simulink model "inv_pendel4"  (Simulink 4.00)
settings: Solver=ode45  StartTime=0.0  StopTime=10.0  MaxStep=0.01  RelTol=1e-3
values from neighbouring files (symbols this model uses):
  g = 9.89    [inv_pendel_1.m]    (also in inv_pendel_2.m; inv_pendel_3.m; inv_pendel_4.m)
  K = place(a,b,p)    [inv_pendel_2.m]    (also in inv_pendel_3.m; inv_pendel_4.m; zeitdiskret_1.m = [1,0;10,1])
  l = 0.75    [inv_pendel_1.m]    (also in inv_pendel_2.m; inv_pendel_3.m; inv_pendel_4.m)
  M = 5    [inv_pendel_1.m]    (also in inv_pendel_2.m; inv_pendel_3.m; inv_pendel_4.m)
  m = 0.5    [inv_pendel_1.m]    (also in inv_pendel_2.m; inv_pendel_3.m; inv_pendel_4.m; mikrofon1.m = 0.001)
libraries: cstblocks x2
settings Model: LastModifiedBy=Administrator  BlockReductionOpt=off

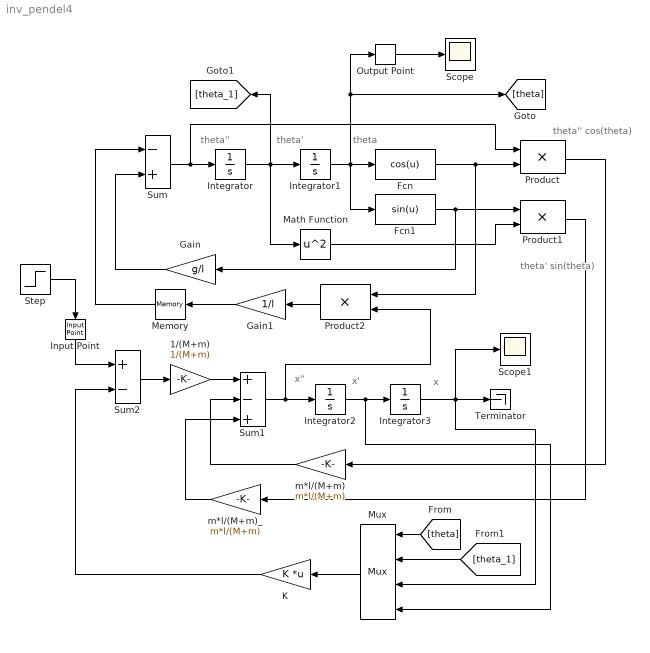
== system inv_pendel4 ==
  note: theta''
  note: theta'
  note: theta
  note: theta'' cos(theta)
  note: theta' sin(theta)
  note: x''
  note: x'
  note: x
  1/(M+m) : Gain  Gain=1/(M+m)  Multiplication=Element-wise(K.*u)  SaturateOnIntegerOverflow=on
  Fcn : Fcn  Expr=cos(u)
  Fcn1 : Fcn  Expr=sin(u)
  Gain : Gain  Orientation=left  Gain=g/l  Multiplication=Element-wise(K.*u)  SaturateOnIntegerOverflow=on
  Gain1 : Gain  Orientation=left  Gain=1/l  Multiplication=Element-wise(K.*u)  SaturateOnIntegerOverflow=on
  Input Point : cstblocks/Input Point  Orientation=down
  Integrator : Integrator  ExternalReset=none  InitialConditionSource=internal  InitialCondition=0  LimitOutput=off  UpperSaturationLimit=inf  LowerSaturationLimit=-inf  ShowSaturationPort=off  ShowStatePort=off  AbsoluteTolerance=auto
  Integrator1 : Integrator  ExternalReset=none  InitialConditionSource=internal  InitialCondition=0.2  LimitOutput=off  UpperSaturationLimit=inf  LowerSaturationLimit=-inf  ShowSaturationPort=off  ShowStatePort=off  AbsoluteTolerance=auto
  Integrator2 : Integrator  ExternalReset=none  InitialConditionSource=internal  InitialCondition=0  LimitOutput=off  UpperSaturationLimit=inf  LowerSaturationLimit=-inf  ShowSaturationPort=off  ShowStatePort=off  AbsoluteTolerance=auto
  Integrator3 : Integrator  ExternalReset=none  InitialConditionSource=internal  InitialCondition=0  LimitOutput=off  UpperSaturationLimit=inf  LowerSaturationLimit=-inf  ShowSaturationPort=off  ShowStatePort=off  AbsoluteTolerance=auto
  K : Gain  Orientation=left  Gain=K  Multiplication=Matrix(K*u)  SaturateOnIntegerOverflow=on
  Math Function : Math  Operator=square  OutputSignalType=auto
  Memory : Memory  Orientation=left  X0=0  InheritSampleTime=off
  Mux : Mux  Orientation=left  Inputs=4
      settings: DisplayOption=none
  Output Point : cstblocks/Output Point
  Product : Product  Inputs=2  Multiplication=Element-wise(.*)  SaturateOnIntegerOverflow=on
  Product1 : Product  Inputs=2  Multiplication=Element-wise(.*)  SaturateOnIntegerOverflow=on
  Product2 : Product  Orientation=left  Inputs=2  Multiplication=Element-wise(.*)  SaturateOnIntegerOverflow=on
  Scope : Scope
      settings: TimeRange=auto  YMin=-1  YMax=1  SaveToWorkspace=off  SaveName=ScopeData  MaxDataPoints=5000
  Scope1 : Scope
      settings: TimeRange=auto  YMin=-1  YMax=4  SaveToWorkspace=off  MaxDataPoints=5000
  Step : Step  Time=0  Before=0  After=1  SampleTime=0
  Sum : Sum  Inputs=-+  SaturateOnIntegerOverflow=on
  Sum1 : Sum  Inputs=+-+  SaturateOnIntegerOverflow=on
  Sum2 : Sum  Inputs=+-  SaturateOnIntegerOverflow=on
  Terminator : Terminator
  m*l/(M+m) : Gain  Orientation=left  Gain=m*l/(M+m)  Multiplication=Element-wise(K.*u)  SaturateOnIntegerOverflow=on
  m*l/(M+m)_ : Gain  Orientation=left  Gain=m*l/(M+m)  Multiplication=Element-wise(K.*u)  SaturateOnIntegerOverflow=on
  wires:
  Sum/1 -> Integrator/1, Product/1
  Integrator/1 -> Integrator1/1, [theta_1], Math Function/1
  Integrator1/1 -> Fcn1/1, Fcn/1, [theta], Output Point/1
  Fcn/1 -> Product2/1, Product/2
  Fcn1/1 -> Product1/1, Gain/1
  Product/1 -> m*l/(M+m)/1
  Gain/1 -> Sum/2
  Product2/1 -> Gain1/1
  Gain1/1 -> Memory/1
  Sum1/1 -> Integrator2/1, Product2/2
  Integrator2/1 -> Integrator3/1, Mux/4
  1/(M+m)/1 -> Sum1/1
  m*l/(M+m)/1 -> Sum1/2
  m*l/(M+m)_/1 -> Sum1/3
  Product1/1 -> m*l/(M+m)_/1
  Integrator3/1 -> Terminator/1, Scope1/1, Mux/3
  Sum2/1 -> 1/(M+m)/1
  Mux/1 -> K/1
  [theta] -> Mux/1
  [theta_1] -> Mux/2
  Math Function/1 -> Product1/2
  Step/1 -> Input Point/1
  Input Point/1 -> Sum2/1
  Output Point/1 -> Scope/1
  K/1 -> Sum2/2
  Memory/1 -> Sum/1
